simulink model "Steer_example"  (Simulink 8.3)
settings: Solver=ode45  StartTime=0.0  StopTime=25  RelTol=1e-3
libraries: Solver_SF x1
settings Model: Creator=msayers  LastModifiedBy=AK-47
settings DataIOCC: SignalLoggingName=sigsOut
settings OptimizationCC: ExpressionDepthLimit=2147483647  InitFltsAndDblsToZero=on
settings DebuggingCC: SaveWithParameterizedLinksMsg=none  SignalResolutionControl=TryResolveAllWithWarning  SolverPrmCheckMsg=none  MultiTaskDSMMsg=warning  MultiTaskCondExecSysMsg=none  FcnCallInpInsideContextMsg=UseLocalSettings
settings HardwareCC: TargetUnknown=on
settings RTWCC: IncludeERTFirstTime=on
settings GRTTargetCC: TargetFcnLib=ansi_tfl_tmw.mat

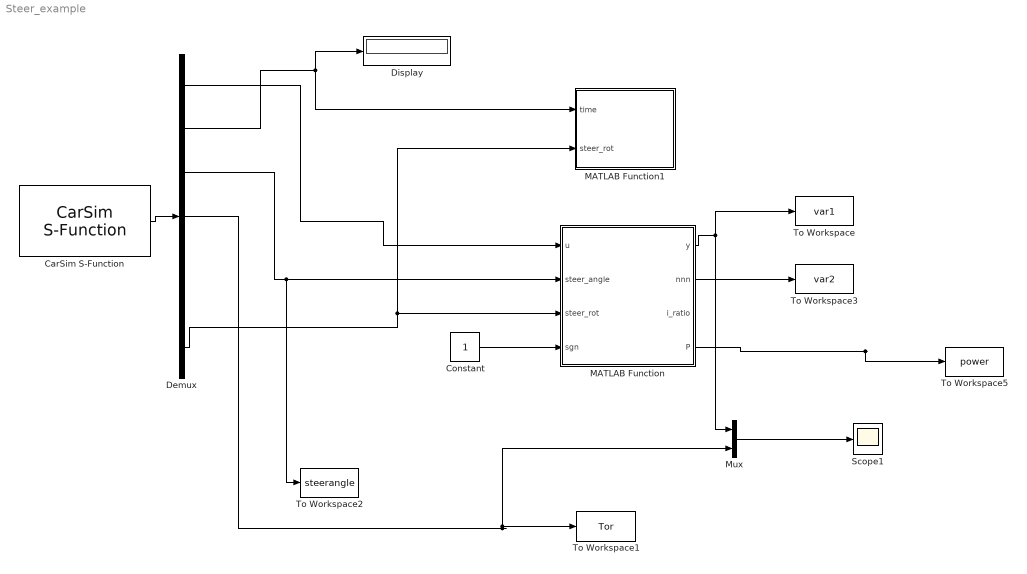
== system Steer_example ==
  CarSim S-Function : Solver_SF/CarSim S-Function  Priority=1  VehicleCode=i_i  SIMFILE=simfile.sim
  Constant : Constant
  Demux : Demux  Outputs="[1 1 1 1 1 1 1  ]"
  Display : Display
  MATLAB Function : MATLAB Function  TreatAsAtomicUnit=on
  MATLAB Function1 : MATLAB Function  TreatAsAtomicUnit=on
  Mux : Mux  Inputs=2
  Scope1 : Scope
      settings: ShowLegends=on
  To Workspace : ToWorkspace  VariableName=var1  SampleTime=-1
  To Workspace1 : ToWorkspace  VariableName=Tor  SampleTime=-1
  To Workspace2 : ToWorkspace  VariableName=steerangle  SampleTime=-1
  To Workspace3 : ToWorkspace  VariableName=var2  SampleTime=-1
  To Workspace5 : ToWorkspace  VariableName=power  SampleTime=-1
  wires:
  CarSim S-Function/1 -> Demux/1
  MATLAB Function/1(y) -> Mux/1, To Workspace/1
  Demux/1 -> MATLAB Function/1(u)
  Demux/7 -> MATLAB Function1/2(steer_rot), MATLAB Function/3(steer_rot)
  MATLAB Function/2(nnn) -> To Workspace3/1
  Demux/3 -> MATLAB Function/2(steer_angle), To Workspace2/1
  Demux/4 -> Mux/2, To Workspace1/1
  Mux/1 -> Scope1/1
  Constant/1 -> MATLAB Function/4(sgn)
  Demux/2 -> MATLAB Function1/1(time), Display/1
  MATLAB Function/4(P) -> To Workspace5/1

== matlab function MATLAB Function1 ==
  data: time input double; steer_rot input double

function   fcn(time,steer_rot)
coder.extrinsic('set_param')
if(time < .01)
     if(steer_rot > 0)
     set_param('Steer_example/Constant','Value','1')
     else
         set_param('Steer_example/Constant','Value','-1')
     end

end

== matlab function MATLAB Function ==
  data: u input double; y output double; steer_angle input double; nnn output double; steer_rot input double; i_ratio output double; sgn input double; P output double
function [y,nnn,i_ratio,P] = fcn(u,steer_angle,steer_rot,sgn)
m = 1818.2;
a = 1.463;
b = 1.585;
I = 3885;
kf = 95000;
kr = 90000;
G = .284;
N1 = 16;
N2 = 20;
mu1 = .94;
mu2 = .90;
tptm = .05;
K = (m/((a+b)^2))*((a/kr) - (b/kf));
nnn = N1*steer_rot;

if(u <= 20)
     i = 7;
elseif(u >= 100)
     i = 25;
else
     i = (u/(a+b))/(G * (1 + K*(u^2)));
end
 
i_ratio = i;
p1 = kf*(tptm);
p2 = mu1*mu2*N1*N2;
p3 = a+b+((m*a*(u^2))/(kr*(a+b)));
p4 = 1 + (K*(u^2));
p5 = steer_angle/i;
T = (p1/p2)*(((p3)/(p4))-1)*p5;
if(sgn > 0)
y = T/1000;
else
  y = -T/1000;
end
P = abs(y)*1000*abs(nnn)*(pi/180);
